simulink model "q_five"  (R2019b)
settings: Solver=VariableStepAuto  StartTime=0.0  StopTime=10  RelTol=1e-3
values from neighbouring files (symbols this model uses):
  A_fs = [-0.5 0 -455;0 -2.9 455; 1 -1 0]    [ex4.m]    (also in ex5.m; ex5test.m)
  B_fs = [17 0; 0 -5; 0 0]    [ex4.m]    (also in ex5.m; ex5test.m)
  C_fs = [1 0 0; 0 1 0; 0 0 1]    [ex4.m]    (also in ex5.m; ex5test.m)
  D_fs = [0 0;0 0; 0 0]    [ex4.m]    (also in ex5.m; ex5test.m)
  kq4 = place(A4, B4, p4)    [ex4.m]    (also in ex5.m; ex5test.m)
  L = [2253.1; 246.6; 57.5]    [ex5.m]    (also in ex5test.m = Tinv*L0)
settings Model: Creator=kecy6rkk  LastModifiedBy=rafek
settings SFSimCC: CustomCodeUndefinedFunction=UseInterfaceOnly

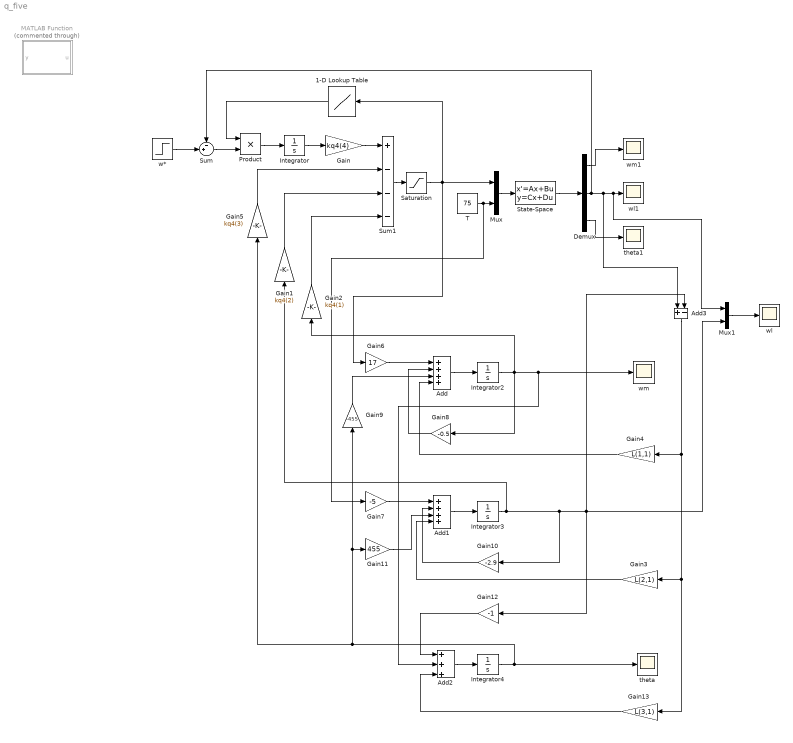
== system q_five ==
  1-D Lookup Table : Lookup_n-D  NumberOfTableDimensions=1  BreakpointsForDimension1=[-100, -32, -31.9, 0, 31.9, 32, 100]  Table=[0, 0, 1, 1, 1, 0, 0]  InternalRulePriority=Speed  RndMeth=Simplest  InputSameDT=on
  Add : Sum  Inputs=++++
  Add1 : Sum  Inputs=++++
  Add2 : Sum  Inputs=+++
  Add3 : Sum  Inputs=+-
  Demux : Demux  Outputs=3
  Gain : Gain  Gain=kq4(4)
  Gain1 : Gain  Gain=kq4(2)
  Gain10 : Gain  Gain=-2.9
  Gain11 : Gain  Gain=455
  Gain12 : Gain  Gain=-1
  Gain13 : Gain  Gain=L(3,1)
  Gain2 : Gain  Gain=kq4(1)
  Gain3 : Gain  Gain=L(2,1)
  Gain4 : Gain  Gain=L(1,1)
  Gain5 : Gain  Gain=kq4(3)
  Gain6 : Gain  Gain=17
  Gain7 : Gain  Gain=-5
  Gain8 : Gain  Gain=-0.5
  Gain9 : Gain  Gain=-455
  Integrator{,2..4} (4 alike) : Integrator
  MATLAB Function : MATLAB Function  Commented=through  TreatAsAtomicUnit=on
  Mux : Mux  Inputs=2
  Mux1 : Mux  Inputs=2
  Product : Product
  Saturation : Saturate  UpperLimit=32  LowerLimit=-32
  State-Space : StateSpace  A=A_fs  B=B_fs  C=C_fs  D=D_fs  InitialCondition=0
  Sum : Sum  Inputs=-+|
  Sum1 : Sum  Inputs=+---
  T : Constant  Value=75
  theta : Scope
  theta1 : Scope
  w* : Step  Time=0  After=100  SampleTime=0
  wl : Scope
  wl1 : Scope
  wm : Scope
  "wm1 " : Scope
  wires:
  Gain/1 -> Sum1/1
  Integrator/1 -> Gain/1
  T/1 -> Gain7/1, Mux/2
  Mux/1 -> State-Space/1
  State-Space/1 -> Demux/1
  Demux/1 -> "wm1 "/1
  Demux/2 -> Mux1/1, wl1/1, Add3/1, Sum/1
  Demux/3 -> theta1/1
  Gain5/1 -> Sum1/2
  w*/1 -> Sum/2
  Integrator4/1 -> theta/1, Gain5/1, Gain11/1, Gain9/1
  Add2/1 -> Integrator4/1
  Add1/1 -> Integrator3/1
  Gain8/1 -> Add/2
  Gain6/1 -> Add/1
  Integrator3/1 -> Gain10/1, Add3/2, Mux1/2, Gain12/1, Gain1/1
  Integrator2/1 -> Gain2/1, wm/1, Add2/2, Gain8/1
  Gain7/1 -> Add1/1
  Add/1 -> Integrator2/1
  Gain10/1 -> Add1/2
  Gain9/1 -> Add/3
  Gain11/1 -> Add1/3
  Gain12/1 -> Add2/1
  Add3/1 -> Gain4/1, Gain13/1, Gain3/1
  Gain3/1 -> Add1/4
  Gain4/1 -> Add/4
  Gain13/1 -> Add2/3
  Gain2/1 -> Sum1/4
  Gain1/1 -> Sum1/3
  Sum/1 -> Product/2
  Product/1 -> Integrator/1
  1-D Lookup Table/1 -> Product/1
  Sum1/1 -> Saturation/1
  Saturation/1 -> 1-D Lookup Table/1, Gain6/1, Mux/1
  Mux1/1 -> wl/1

== matlab function q_five/MATLAB Function ==
  data: u input; y output
function y = fcn(u)
if u>42 || u<0
    y=0;
else
    y=1;
end
end
